simulink model "DiscreteIntegrator_TestGen10"  (R2017b)
settings: Solver=FixedStepDiscrete  StartTime=0.0  StopTime=10.0  RelTol=1e-3
undefined symbols (not defined in the file): DiscIntNeverNeededParam
settings Model: Creator=hbourbou  LastModifiedBy=hbourbou
settings DebuggingCC: ParameterOverflowMsg=none

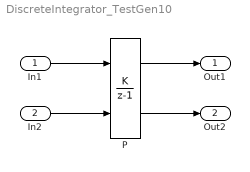
== system DiscreteIntegrator_TestGen10 ==
  In1 : Inport  OutDataTypeStr=int16  PortDimensions=1
  In2 : Inport  Port=2
  P : DiscreteIntegrator  IntegratorMethod=Accumulation: Forward Euler  gainval=2.0  InitialConditionSource=external  InitialCondition=7  SampleTime=-1  OutDataTypeStr=int16  SaturateOnIntegerOverflow=on  LimitOutput=on  UpperSaturationLimit=100  LowerSaturationLimit=5  ShowSaturationPort=on  ICPrevOutput=DiscIntNeverNeededParam  ICPrevScaledInput=DiscIntNeverNeededParam
  Out1 : Outport
  Out2 : Outport  Port=2
  wires:
  In1/1 -> P/1
  In2/1 -> P/2
  P/1 -> Out1/1
  P/2 -> Out2/1
